simulink model "latest_coil"  (R2021b)
settings: Solver=FixedStepAuto  StartTime=-8e-3  StopTime=8e-3  FixedStep=1e-4  RelTol=1e-3
undefined symbols (not defined in the file or in its folder): X, Y, Z
libraries: sm_lib x15, nesl_utility x1
(part 1 of 2)
settings Model: Creator=teja  LastModifiedBy=teja

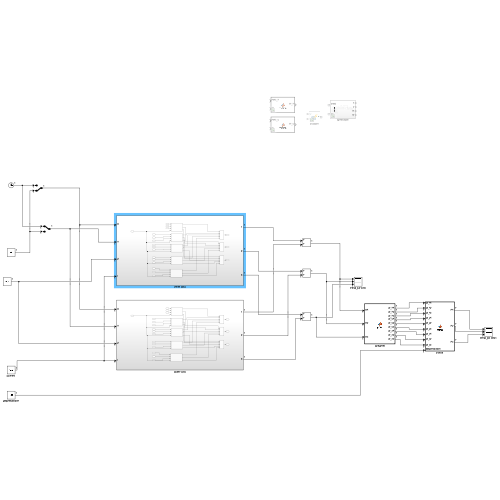
[thumbnail: Simulink's stored preview of the top-level diagram]
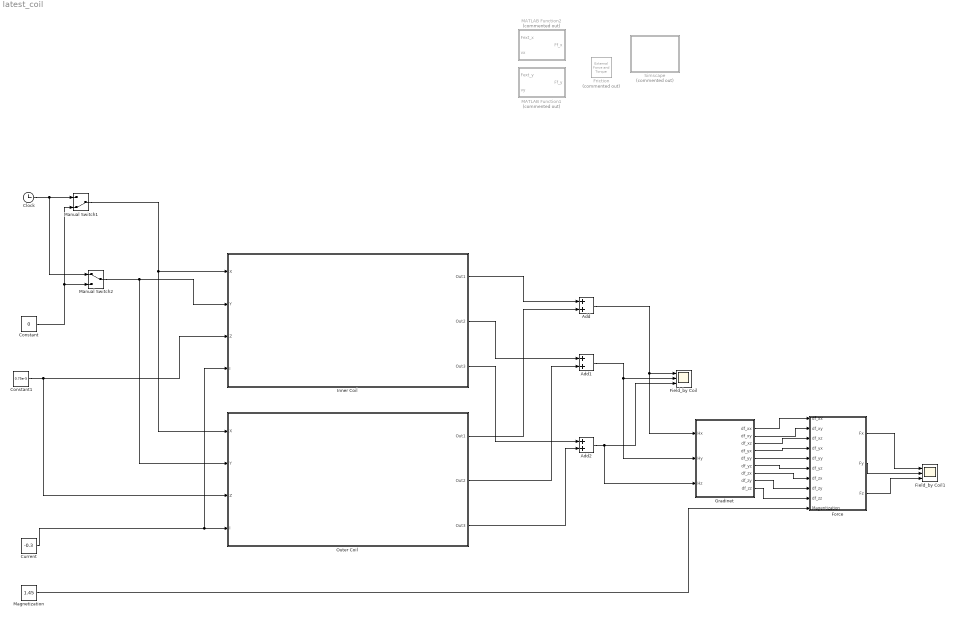
== system latest_coil ==
  Add : Sum
  Add1 : Sum
  Add2 : Sum
  Clock : Clock
  Constant : Constant  Value=0
  Constant1 : Constant  Value=0.75e-5
  Current : Constant  Value=-0.3
  Field_by Coil : Scope  NumInputPorts=3
  Field_by Coil1 : Scope  NumInputPorts=3
  Force : MATLAB Function  TreatAsAtomicUnit=on
  Friction : sm_lib/Forces and Torques/External Force and Torque  Commented=on  ForceResolutionFrame=World  EnableForceX=on  EnableForceY=on  EnableForceZ=off  EnableForce=off  TorqueResolutionFrame=AttachedFrame  EnableTorqueX=off  EnableTorqueY=off  EnableTorqueZ=off  EnableTorque=off
  Gradinet : MATLAB Function  TreatAsAtomicUnit=on
  Inner Coil : Subsystem
  MATLAB Function1 : MATLAB Function  Commented=on  TreatAsAtomicUnit=on
  MATLAB Function2 : MATLAB Function  Commented=on  TreatAsAtomicUnit=on
  Magnetization : Constant  Value=1.45
  Manual Switch1 : ManualSwitch  CurrentSetting=0
  Manual Switch2 : ManualSwitch
  Outer Coil : Subsystem
  Simscape : Subsystem  Commented=on
  wires:
  Constant/1 -> Manual Switch2/2, Manual Switch1/2
  Constant1/1 -> Outer Coil/3(Z), Inner Coil/3(Z)
  Current/1 -> Outer Coil/4(I), Inner Coil/4(I)
  Inner Coil/1(Out1) -> Add/1
  Outer Coil/1(Out1) -> Add/2
  Inner Coil/2(Out2) -> Add1/1
  Outer Coil/2(Out2) -> Add1/2
  Inner Coil/3(Out3) -> Add2/1
  Outer Coil/3(Out3) -> Add2/2
  Add2/1 -> Gradinet/3(Hz), Field_by Coil/3
  Add1/1 -> Gradinet/2(Hy), Field_by Coil/2
  Add/1 -> Gradinet/1(Hx), Field_by Coil/1
  Manual Switch1/1 -> Outer Coil/1(X), Inner Coil/1(X)
  Clock/1 -> Manual Switch2/1, Manual Switch1/1
  Manual Switch2/1 -> Outer Coil/2(Y), Inner Coil/2(Y)
  Gradinet/1(df_xx) -> Force/1(df_xx)
  Gradinet/2(df_xy) -> Force/2(df_xy)
  Gradinet/3(df_xz) -> Force/3(df_xz)
  Gradinet/4(df_yx) -> Force/4(df_yx)
  Gradinet/5(df_yy) -> Force/5(df_yy)
  Gradinet/6(df_yz) -> Force/6(df_yz)
  Gradinet/7(df_zx) -> Force/7(df_zx)
  Gradinet/8(df_zy) -> Force/8(df_zy)
  Gradinet/9(df_zz) -> Force/9(df_zz)
  Force/1(Fx) -> Field_by Coil1/1
  Force/2(Fy) -> Field_by Coil1/2
  Force/3(Fz) -> Field_by Coil1/3
  Magnetization/1 -> Force/10(Magentization)

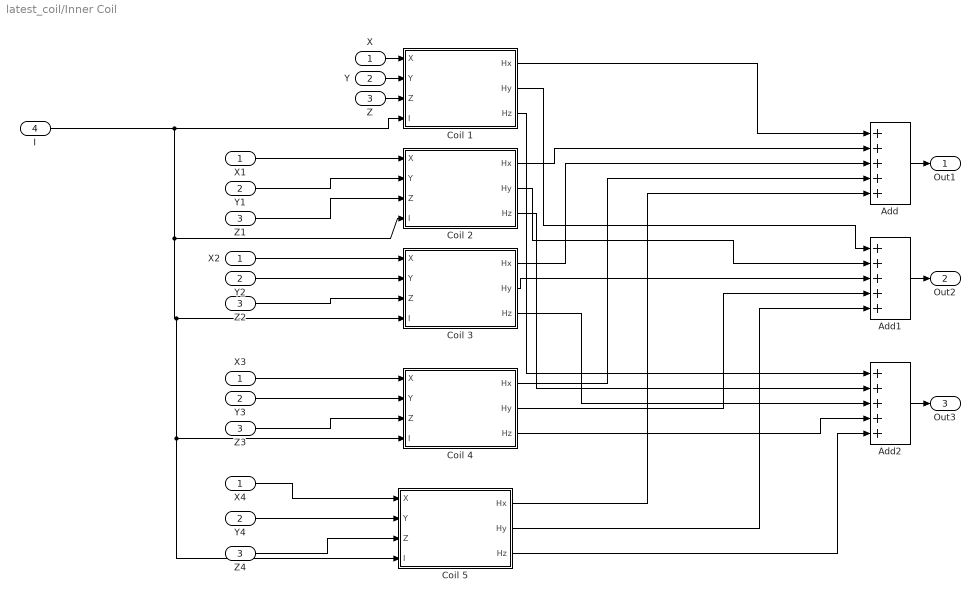
== system latest_coil/Inner Coil ==
  X : Inport
  Y : Inport  Port=2
  Z : Inport  Port=3
  I : Inport  Port=4
  Add : Sum  Inputs=+++++
  Add1 : Sum  Inputs=+++++
  Add2 : Sum  Inputs=+++++
  Coil 1 : Subsystem
  Coil 2 : Subsystem
  Coil 3 : Subsystem
  Coil 4 : Subsystem
  Coil 5 : Subsystem
  X{1..4} (4 alike) : InportShadow
  Y{1..4} (4 alike) : InportShadow  Port=2
  Z{1..4} (4 alike) : InportShadow  Port=3
  Out1 : Outport
  Out2 : Outport  Port=2
  Out3 : Outport  Port=3
  wires:
  Y/1 -> Coil 1/2(Y)
  Coil 2/2(Hy) -> Add1/2
  Add2/1 -> Out3/1
  Z/1 -> Coil 1/3(Z)
  Add1/1 -> Out2/1
  Z1/1 -> Coil 2/3(Z)
  Add/1 -> Out1/1
  Coil 4/2(Hy) -> Add1/4
  Y2/1 -> Coil 3/2(Y)
  Z2/1 -> Coil 3/3(Z)
  Coil 1/1(Hx) -> Add/1
  X4/1 -> Coil 5/1(X)
  Coil 3/2(Hy) -> Add1/3
  I/1 -> Coil 1/4(I), Coil 5/4(I), Coil 4/4(I), Coil 3/4(I), Coil 2/4(I)
  Coil 3/1(Hx) -> Add/3
  X1/1 -> Coil 2/1(X)
  Z4/1 -> Coil 5/3(Z)
  Coil 2/3(Hz) -> Add2/2
  Coil 5/2(Hy) -> Add1/5
  Coil 4/1(Hx) -> Add/4
  X3/1 -> Coil 4/1(X)
  Coil 1/2(Hy) -> Add1/1
  Coil 2/1(Hx) -> Add/2
  Z3/1 -> Coil 4/3(Z)
  Coil 5/1(Hx) -> Add/5
  Coil 3/3(Hz) -> Add2/3
  Coil 5/3(Hz) -> Add2/5
  Y4/1 -> Coil 5/2(Y)
  X/1 -> Coil 1/1(X)
  Coil 4/3(Hz) -> Add2/4
  X2/1 -> Coil 3/1(X)
  Y3/1 -> Coil 4/2(Y)
  Coil 1/3(Hz) -> Add2/1
  Y1/1 -> Coil 2/2(Y)

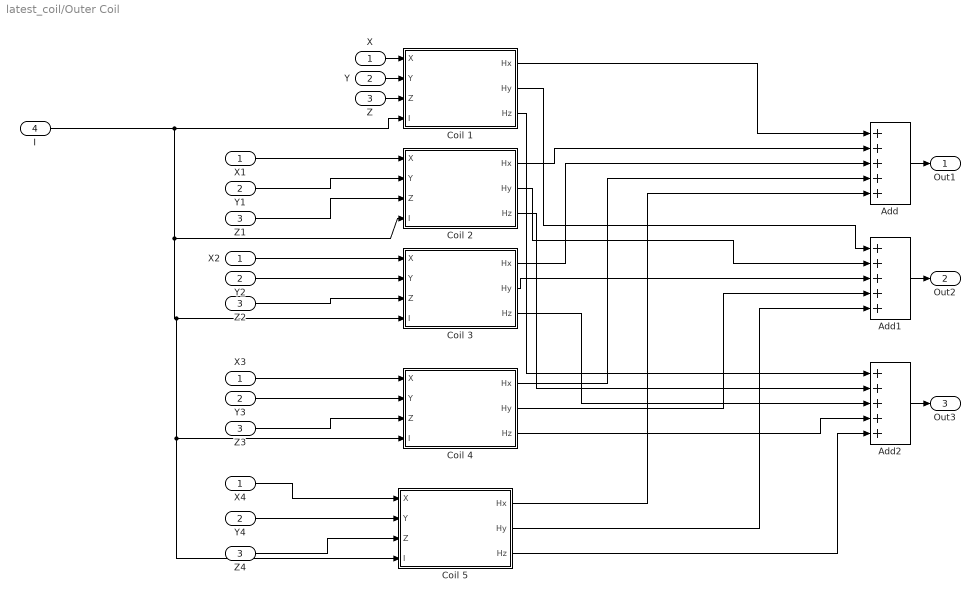
== system latest_coil/Outer Coil ==
  X : Inport
  Y : Inport  Port=2
  Z : Inport  Port=3
  I : Inport  Port=4
  Add : Sum  Inputs=+++++
  Add1 : Sum  Inputs=+++++
  Add2 : Sum  Inputs=+++++
  Coil 1 : Subsystem
  Coil 2 : Subsystem
  Coil 3 : Subsystem
  Coil 4 : Subsystem
  Coil 5 : Subsystem
  X{1..4} (4 alike) : InportShadow
  Y{1..4} (4 alike) : InportShadow  Port=2
  Z{1..4} (4 alike) : InportShadow  Port=3
  Out1 : Outport
  Out2 : Outport  Port=2
  Out3 : Outport  Port=3
  wires:
  Y1/1 -> Coil 2/2(Y)
  Coil 1/3(Hz) -> Add2/1
  Y3/1 -> Coil 4/2(Y)
  X2/1 -> Coil 3/1(X)
  Coil 4/3(Hz) -> Add2/4
  X/1 -> Coil 1/1(X)
  Y4/1 -> Coil 5/2(Y)
  Coil 5/3(Hz) -> Add2/5
  Coil 3/3(Hz) -> Add2/3
  Coil 5/1(Hx) -> Add/5
  Z3/1 -> Coil 4/3(Z)
  Coil 2/1(Hx) -> Add/2
  Coil 1/2(Hy) -> Add1/1
  X3/1 -> Coil 4/1(X)
  Coil 4/1(Hx) -> Add/4
  Coil 5/2(Hy) -> Add1/5
  Coil 2/3(Hz) -> Add2/2
  Z4/1 -> Coil 5/3(Z)
  X1/1 -> Coil 2/1(X)
  Coil 3/1(Hx) -> Add/3
  I/1 -> Coil 2/4(I), Coil 3/4(I), Coil 4/4(I), Coil 5/4(I), Coil 1/4(I)
  Coil 3/2(Hy) -> Add1/3
  X4/1 -> Coil 5/1(X)
  Coil 1/1(Hx) -> Add/1
  Z2/1 -> Coil 3/3(Z)
  Y2/1 -> Coil 3/2(Y)
  Coil 4/2(Hy) -> Add1/4
  Add/1 -> Out1/1
  Z1/1 -> Coil 2/3(Z)
  Add1/1 -> Out2/1
  Z/1 -> Coil 1/3(Z)
  Add2/1 -> Out3/1
  Coil 2/2(Hy) -> Add1/2
  Y/1 -> Coil 1/2(Y)

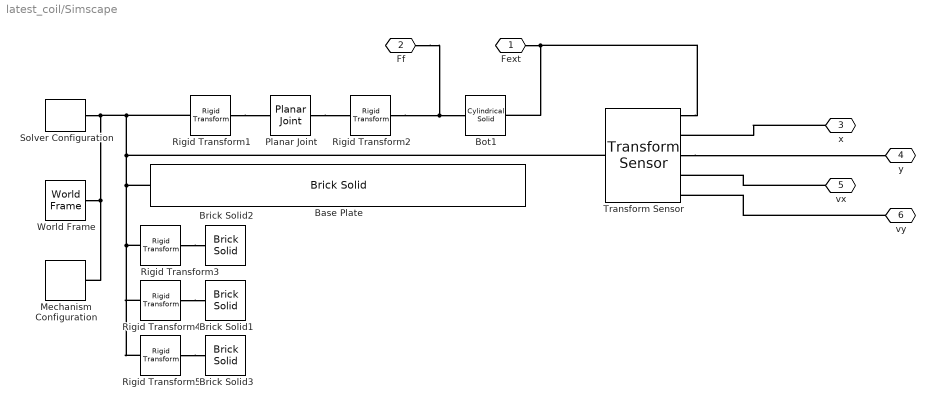
== system latest_coil/Simscape ==
  Base Plate : sm_lib/Body Elements/Brick Solid  GraphicAmbientColor=[0.15 0.15 0.15 1.0]  BasedOnType=Density  BrickDimensions=[100 100 0.15]  BrickDimensionUnits=mm  CenterOfMass=[0 0 0]  CenterOfMassUnits=m  GraphicDiffuseColor=[0.5 0.5 0.5]  Density=1000  DensityUnits=kg/m^3  DoExposeReferenceFrame=off  GraphicEmissiveColor=[0.0 0.0 0.0 1.0]  ExportEntireGeometry=off  SerializedFrames=<Frames><Frame><Id>Frame1</Id><Value><Name>Top</Name><Origin><Source>GeometricFeature</Source><FeatureName>+z surface</FeatureName></Origin><PrimaryAxis><DefinedDirection>+Z</DefinedDirection><Source>ReferenceFrame</Source><SourceDirection>+Z</SourceDirection><FeatureName></FeatureName></PrimaryAxis><SecondaryAxis><DefinedDirection>+X</DefinedDirection><Source>ReferenceFrame</Source><SourceDirection>+X</SourceDirection><FeatureName></FeatureName></SecondaryAxis></Value></Frame></Frames>  MarkerShape=Sphere  MarkerSize=10  GraphicType=FromGeometry  InertiaType=CalculateFromGeometry  Mass=1  MassUnits=kg  MomentsOfInertia=[1 1 1]  MomentsOfInertiaUnits=kg*m^2  GraphicOpacity=1.0  ProductsOfInertia=[0 0 0]  ProductsOfInertiaUnits=kg*m^2  GraphicShininess=75  GraphicSpecularColor=[0.5 0.5 0.5 1.0]  GraphicVisPropType=SimpleVisualProperties
  Bot1 : sm_lib/Body Elements/Cylindrical Solid  GraphicAmbientColor=[0.15 0.15 0.15 1.0]  BasedOnType=Density  CenterOfMass=[0 0 0]  CenterOfMassUnits=m  GraphicDiffuseColor=[0 0.5 0.5]  CylinderLength=10  CylinderLengthUnits=mm  CylinderRadius=20  CylinderRadiusUnits=mm  Density=7300  DensityUnits=kg/m^3  DoExposeReferenceFrame=on  GraphicEmissiveColor=[0.0 0.0 0.0 1.0]  ExportEntireGeometry=off  SerializedFrames=<Frames><Frame><Id>Frame1</Id><Value><Name>Bottom</Name><Origin><Source>GeometricFeature</Source><FeatureName>bottom surface</FeatureName></Origin><PrimaryAxis><DefinedDirection>+Z</DefinedDirection><Source>ReferenceFrame</Source><SourceDirection>+Z</SourceDirection><FeatureName></FeatureName></PrimaryAxis><SecondaryAxis><DefinedDirection>+X</DefinedDirection><Source>ReferenceFrame</Source><SourceDirection>+X</SourceDirection><FeatureName></FeatureName></SecondaryAxis></Value></Frame></Frames>  MarkerShape=Sphere  MarkerSize=10  GraphicType=FromGeometry  InertiaType=CalculateFromGeometry  Mass=1  MassUnits=kg  MomentsOfInertia=[1 1 1]  MomentsOfInertiaUnits=kg*m^2  GraphicOpacity=1.0  ProductsOfInertia=[0 0 0]  ProductsOfInertiaUnits=kg*m^2  GraphicShininess=75  GraphicSpecularColor=[0.5 0.5 0.5 1.0]  GraphicVisPropType=SimpleVisualProperties
  Brick Solid1 : sm_lib/Body Elements/Brick Solid  GraphicAmbientColor=[0.15 0.15 0.15 1.0]  BasedOnType=Density  BrickDimensions=[8 8 0.5]  BrickDimensionUnits=mm  CenterOfMass=[0 0 0]  CenterOfMassUnits=m  GraphicDiffuseColor=[0.5 0.5 0]  Density=1000  DensityUnits=kg/m^3  DoExposeReferenceFrame=off  GraphicEmissiveColor=[0.0 0.0 0.0 1.0]  ExportEntireGeometry=off  SerializedFrames=<Frames><Frame><Id>Frame1</Id><Value><Name>base</Name><Origin><Source>GeometricFeature</Source><FeatureName>-z surface</FeatureName></Origin><PrimaryAxis><DefinedDirection>+Z</DefinedDirection><Source>ReferenceFrame</Source><SourceDirection>+Z</SourceDirection><FeatureName></FeatureName></PrimaryAxis><SecondaryAxis><DefinedDirection>+X</DefinedDirection><Source>ReferenceFrame</Source><SourceDirection>+X</SourceDirection><FeatureName></FeatureName></SecondaryAxis></Value></Frame></Frames>  MarkerShape=Sphere  MarkerSize=10  GraphicType=FromGeometry  InertiaType=CalculateFromGeometry  Mass=1  MassUnits=kg  MomentsOfInertia=[1 1 1]  MomentsOfInertiaUnits=kg*m^2  GraphicOpacity=1.0  ProductsOfInertia=[0 0 0]  ProductsOfInertiaUnits=kg*m^2  GraphicShininess=75  GraphicSpecularColor=[0.5 0.5 0.5 1.0]  GraphicVisPropType=SimpleVisualProperties
  Brick Solid2 : sm_lib/Body Elements/Brick Solid  GraphicAmbientColor=[0.15 0.15 0.15 1.0]  BasedOnType=Density  BrickDimensions=[8 8 0.5]  BrickDimensionUnits=mm  CenterOfMass=[0 0 0]  CenterOfMassUnits=m  GraphicDiffuseColor=[0.5 0.5 0]  Density=1000  DensityUnits=kg/m^3  DoExposeReferenceFrame=off  GraphicEmissiveColor=[0.0 0.0 0.0 1.0]  ExportEntireGeometry=off  SerializedFrames=<Frames><Frame><Id>Frame1</Id><Value><Name>base</Name><Origin><Source>GeometricFeature</Source><FeatureName>-z surface</FeatureName></Origin><PrimaryAxis><DefinedDirection>+Z</DefinedDirection><Source>ReferenceFrame</Source><SourceDirection>+Z</SourceDirection><FeatureName></FeatureName></PrimaryAxis><SecondaryAxis><DefinedDirection>+X</DefinedDirection><Source>ReferenceFrame</Source><SourceDirection>+X</SourceDirection><FeatureName></FeatureName></SecondaryAxis></Value></Frame></Frames>  MarkerShape=Sphere  MarkerSize=10  GraphicType=FromGeometry  InertiaType=CalculateFromGeometry  Mass=1  MassUnits=kg  MomentsOfInertia=[1 1 1]  MomentsOfInertiaUnits=kg*m^2  GraphicOpacity=1.0  ProductsOfInertia=[0 0 0]  ProductsOfInertiaUnits=kg*m^2  GraphicShininess=75  GraphicSpecularColor=[0.5 0.5 0.5 1.0]  GraphicVisPropType=SimpleVisualProperties
  Brick Solid3 : sm_lib/Body Elements/Brick Solid  GraphicAmbientColor=[0.15 0.15 0.15 1.0]  BasedOnType=Density  BrickDimensions=[8 8 0.5]  BrickDimensionUnits=mm  CenterOfMass=[0 0 0]  CenterOfMassUnits=m  GraphicDiffuseColor=[0.5 0.5 0]  Density=1000  DensityUnits=kg/m^3  DoExposeReferenceFrame=off  GraphicEmissiveColor=[0.0 0.0 0.0 1.0]  ExportEntireGeometry=off  SerializedFrames=<Frames><Frame><Id>Frame1</Id><Value><Name>base</Name><Origin><Source>GeometricFeature</Source><FeatureName>-z surface</FeatureName></Origin><PrimaryAxis><DefinedDirection>+Z</DefinedDirection><Source>ReferenceFrame</Source><SourceDirection>+Z</SourceDirection><FeatureName></FeatureName></PrimaryAxis><SecondaryAxis><DefinedDirection>+X</DefinedDirection><Source>ReferenceFrame</Source><SourceDirection>+X</SourceDirection><FeatureName></FeatureName></SecondaryAxis></Value></Frame></Frames>  MarkerShape=Sphere  MarkerSize=10  GraphicType=FromGeometry  InertiaType=CalculateFromGeometry  Mass=1  MassUnits=kg  MomentsOfInertia=[1 1 1]  MomentsOfInertiaUnits=kg*m^2  GraphicOpacity=1.0  ProductsOfInertia=[0 0 0]  ProductsOfInertiaUnits=kg*m^2  GraphicShininess=75  GraphicSpecularColor=[0.5 0.5 0.5 1.0]  GraphicVisPropType=SimpleVisualProperties
  Mechanism Configuration : sm_lib/Utilities/Mechanism Configuration  UniformGravity=Constant  GravityVector=[0 0 -9.80665]  GravityUnits=m/s^2  LinearizationDelta=0.001  JointModeTransitionNonlinearIterations=2
  Planar Joint : sm_lib/Joints/Planar Joint  JointMode=Normal  SenseConstraintForce=off  SenseConstraintForceX=off  SenseConstraintForceY=off  SenseConstraintForceZ=off  SenseConstraintTorque=off  SenseConstraintTorqueX=off  SenseConstraintTorqueY=off  SenseConstraintTorqueZ=off  SenseTotalForce=off  SenseTotalForceX=off  SenseTotalForceY=off  SenseTotalForceZ=off  SenseTotalTorque=off  SenseTotalTorqueX=off  SenseTotalTorqueY=off  SenseTotalTorqueZ=off  CompositeWrenchDir=FollowerOnBase  CompositeWrenchFrame=BaseFrame  PxEquilibriumPosition=0  PxEquilibriumPositionUnits=m  PxSpringStiffness=0  PxSpringStiffnessUnits=N/m  PxDampingCoefficient=0  PxDampingCoefficientUnits=N/(m/s)  PxTorqueActuationMode=NoTorque  PxMotionActuationMode=ComputedMotion  PxSensePosition=off  PxSenseVelocity=off  PxSenseAcceleration=off  PxSenseTorqueForce=off  PxSenseLowerLimitTorqueForce=off  PxSenseUpperLimitTorqueForce=off  PxLowerLimitSpecify=off  PxLowerLimitBound=-1  PxLowerLimitBoundUnits=m  PxLowerLimitStiffness=1e6  PxLowerLimitStiffnessUnits=N/m  PxLowerLimitDamping=1e3  PxLowerLimitDampingUnits=N/(m/s)  PxLowerLimitTransitionRegionWidth=1e-4  PxLowerLimitTransitionRegionWidthUnits=m  PxUpperLimitSpecify=off  PxUpperLimitBound=1  PxUpperLimitBoundUnits=m  PxUpperLimitStiffness=1e6  PxUpperLimitStiffnessUnits=N/m  PxUpperLimitDamping=1e3  PxUpperLimitDampingUnits=N/(m/s)  PxUpperLimitTransitionRegionWidth=1e-4  PxUpperLimitTransitionRegionWidthUnits=m  PxPositionTargetSpecify=off  PxPositionTargetPriority=High  PxPositionTargetValue=0  PxPositionTargetValueUnits=m  PxVelocityTargetSpecify=off  PxVelocityTargetPriority=High  PxVelocityTargetValue=0  PxVelocityTargetValueUnits=m/s  PyEquilibriumPosition=0  PyEquilibriumPositionUnits=m  PySpringStiffness=0  PySpringStiffnessUnits=N/m  PyDampingCoefficient=0  PyDampingCoefficientUnits=N/(m/s)  PyTorqueActuationMode=NoTorque  PyMotionActuationMode=ComputedMotion  PySensePosition=off  PySenseVelocity=off  PySenseAcceleration=off  PySenseTorqueForce=off  PySenseLowerLimitTorqueForce=off  PySenseUpperLimitTorqueForce=off  PyLowerLimitSpecify=off  PyLowerLimitBound=-1  PyLowerLimitBoundUnits=m  PyLowerLimitStiffness=1e6  PyLowerLimitStiffnessUnits=N/m  PyLowerLimitDamping=1e3  PyLowerLimitDampingUnits=N/(m/s)  PyLowerLimitTransitionRegionWidth=1e-4  PyLowerLimitTransitionRegionWidthUnits=m  PyUpperLimitSpecify=off  PyUpperLimitBound=1  PyUpperLimitBoundUnits=m  PyUpperLimitStiffness=1e6  PyUpperLimitStiffnessUnits=N/m  PyUpperLimitDamping=1e3  PyUpperLimitDampingUnits=N/(m/s)  PyUpperLimitTransitionRegionWidth=1e-4  PyUpperLimitTransitionRegionWidthUnits=m  PyPositionTargetSpecify=off  PyPositionTargetPriority=High  PyPositionTargetValue=0  PyPositionTargetValueUnits=m  PyVelocityTargetSpecify=off  PyVelocityTargetPriority=High  PyVelocityTargetValue=0  PyVelocityTargetValueUnits=m/s  RzEquilibriumPosition=0  RzEquilibriumPositionUnits=deg  RzSpringStiffness=0  RzSpringStiffnessUnits=N*m/deg  RzDampingCoefficient=0  RzDampingCoefficientUnits=N*m/(deg/s)  RzTorqueActuationMode=NoTorque  RzMotionActuationMode=ComputedMotion  RzSensePosition=off  RzSenseVelocity=off  RzSenseAcceleration=off  RzSenseTorqueForce=off  RzSenseLowerLimitTorqueForce=off  RzSenseUpperLimitTorqueForce=off  RzLowerLimitSpecify=off  RzLowerLimitBound=-90  RzLowerLimitBoundUnits=deg  RzLowerLimitStiffness=1e4  RzLowerLimitStiffnessUnits=N*m/deg  RzLowerLimitDamping=10  RzLowerLimitDampingUnits=N*m/(deg/s)  RzLowerLimitTransitionRegionWidth=0.1  RzLowerLimitTransitionRegionWidthUnits=deg  RzUpperLimitSpecify=off  RzUpperLimitBound=90  RzUpperLimitBoundUnits=deg  RzUpperLimitStiffness=1e4  RzUpperLimitStiffnessUnits=N*m/deg  RzUpperLimitDamping=10  RzUpperLimitDampingUnits=N*m/(deg/s)  RzUpperLimitTransitionRegionWidth=0.1  RzUpperLimitTransitionRegionWidthUnits=deg  RzPositionTargetSpecify=off  RzPositionTargetPriority=High  RzPositionTargetValue=0  RzPositionTargetValueUnits=deg  RzVelocityTargetSpecify=off  RzVelocityTargetPriority=High  RzVelocityTargetValue=0  RzVelocityTargetValueUnits=deg/s
  Rigid Transform1 : sm_lib/Frames and Transforms/Rigid Transform  TranslationMethod=Cartesian  TranslationStandardOffset=0  TranslationLengthUnit=mm  TranslationStandardAxis=+Z  TranslationCartesianOffset=[0 0 0]  TranslationROffset=0  TranslationROffsetUnits=m  TranslationZOffset=0  TranslationZOffsetUnits=m  TranslationThetaOffset=0  TranslationThetaOffsetUnits=deg  RotationMethod=AlignedAxes  RotationAngleUnits=deg  RotationStandardAxis=+Z  RotationAngle=0.0  RotationArbitraryAxis=[0 0 1]  FollAlignAxisA=+Y  BaseAlignAxisA=+X  FollAlignAxisB=+Z  BaseAlignAxisB=+Z  RotationSequenceAxes=FollowerAxes  RotationSequence=XYX  RotationSequenceAngles=[0 0 0]  RotationSequenceAnglesUnits=deg  RotationMatrix=[1 0 0; 0 1 0; 0 0 1]
  Rigid Transform2 : sm_lib/Frames and Transforms/Rigid Transform  TranslationMethod=None  TranslationStandardOffset=0  TranslationLengthUnit=mm  TranslationStandardAxis=+Z  TranslationCartesianOffset=[-15 0 0.15]  TranslationROffset=0  TranslationROffsetUnits=m  TranslationZOffset=0  TranslationZOffsetUnits=m  TranslationThetaOffset=0  TranslationThetaOffsetUnits=deg  RotationMethod=AlignedAxes  RotationAngleUnits=deg  RotationStandardAxis=+Z  RotationAngle=0.0  RotationArbitraryAxis=[0 0 1]  FollAlignAxisA=+Y  BaseAlignAxisA=+X  FollAlignAxisB=+Z  BaseAlignAxisB=+Z  RotationSequenceAxes=FollowerAxes  RotationSequence=XYX  RotationSequenceAngles=[0 0 0]  RotationSequenceAnglesUnits=deg  RotationMatrix=[1 0 0; 0 1 0; 0 0 1]
  Rigid Transform3 : sm_lib/Frames and Transforms/Rigid Transform  TranslationMethod=Cartesian  TranslationStandardOffset=0  TranslationLengthUnit=mm  TranslationStandardAxis=+Z  TranslationCartesianOffset=[9 0 2]  TranslationROffset=0  TranslationROffsetUnits=m  TranslationZOffset=0  TranslationZOffsetUnits=m  TranslationThetaOffset=0  TranslationThetaOffsetUnits=deg  RotationMethod=None  RotationAngleUnits=deg  RotationStandardAxis=+Z  RotationAngle=0.0  RotationArbitraryAxis=[0 0 1]  FollAlignAxisA=+Y  BaseAlignAxisA=+X  FollAlignAxisB=+Z  BaseAlignAxisB=+Z  RotationSequenceAxes=FollowerAxes  RotationSequence=XYX  RotationSequenceAngles=[0 0 0]  RotationSequenceAnglesUnits=deg  RotationMatrix=[1 0 0; 0 1 0; 0 0 1]
  Rigid Transform4 : sm_lib/Frames and Transforms/Rigid Transform  TranslationMethod=Cartesian  TranslationStandardOffset=0  TranslationLengthUnit=mm  TranslationStandardAxis=+Z  TranslationCartesianOffset=[0 0 2]  TranslationROffset=0  TranslationROffsetUnits=m  TranslationZOffset=0  TranslationZOffsetUnits=m  TranslationThetaOffset=0  TranslationThetaOffsetUnits=deg  RotationMethod=None  RotationAngleUnits=deg  RotationStandardAxis=+Z  RotationAngle=0.0  RotationArbitraryAxis=[0 0 1]  FollAlignAxisA=+Y  BaseAlignAxisA=+X  FollAlignAxisB=+Z  BaseAlignAxisB=+Z  RotationSequenceAxes=FollowerAxes  RotationSequence=XYX  RotationSequenceAngles=[0 0 0]  RotationSequenceAnglesUnits=deg  RotationMatrix=[1 0 0; 0 1 0; 0 0 1]
  Rigid Transform5 : sm_lib/Frames and Transforms/Rigid Transform  TranslationMethod=Cartesian  TranslationStandardOffset=0  TranslationLengthUnit=mm  TranslationStandardAxis=+Z  TranslationCartesianOffset=[-9 0 2]  TranslationROffset=0  TranslationROffsetUnits=m  TranslationZOffset=0  TranslationZOffsetUnits=m  TranslationThetaOffset=0  TranslationThetaOffsetUnits=deg  RotationMethod=None  RotationAngleUnits=deg  RotationStandardAxis=+Z  RotationAngle=0.0  RotationArbitraryAxis=[0 0 1]  FollAlignAxisA=+Y  BaseAlignAxisA=+X  FollAlignAxisB=+Z  BaseAlignAxisB=+Z  RotationSequenceAxes=FollowerAxes  RotationSequence=XYX  RotationSequenceAngles=[0 0 0]  RotationSequenceAnglesUnits=deg  RotationMatrix=[1 0 0; 0 1 0; 0 0 1]
  Solver Configuration : nesl_utility/Solver Configuration  PhysicalDomain=network_engine_domain  SubClassName=solver  LeftPortType=input  RightPortType=generic  Tones=[]  Harmonics=[]  SimulateNoise=off  Profile=off  UseLocalSampling=off  EnableSwitchedLinearOptims=on  FrequencyDomain=off  UseCCode=off  RelTol=0.001  AbsTol=1e-06  MinStep=1e-09  ToWorkspace=off  RevertToSquareIcSolve=off  NumHomotopyIterations=100  PhasorMode=off  PhasorModeNumHarmonics=1  DoDC=off  ResidualTolerance=1e-09  UseLocalSolver=off  LocalSolverChoice=NE_BACKWARD_EULER_ADVANCER  LocalSolverSampleTime=0.001  DoFixedCost=off  MaxNonlinIter=3  MaxModeIter=2  ComputeImpulses=off  ImpulseIterations=2  LinearAlgebra=Sparse  EquationFormulation=NE_TIME_EF  DelaysMemoryBudget=1024  AutomaticFiltering=on  FilteringTimeConstant=0.001  PartitionStorageMethod=AS_NEEDED  PartitionMemoryBudget=1024  PartitionMethod=FAST
      settings: SourceProductBaseCode=PW,SS
  Transform Sensor : sm_lib/Frames and Transforms/Transform Sensor  MeasurementFrame=World  SenseAngle=off  SenseAxis=off  SenseAngle1=off  SenseAngle2=off  SenseAngle3=off  SenseQ=off  SenseR=off  SenseOmegaX=off  SenseOmegaY=off  SenseOmegaZ=off  SenseOmega1=off  SenseOmega2=off  SenseOmega3=off  SenseQDot=off  SenseRDot=off  SenseAlphaX=off  SenseAlphaY=off  SenseAlphaZ=off  SenseAlpha1=off  SenseAlpha2=off  SenseAlpha3=off  SenseQDDot=off  SenseRDDot=off  SenseX=on  SenseY=on  SenseZ=off  SenseRad=off  SenseAzim=off  SenseDist=off  SenseInc=off  SenseXDot=on  SenseYDot=on  SenseZDot=off  SenseRadDot=off  SenseAzimDot=off  SenseDistDot=off  SenseIncDot=off  SenseXDDot=off  SenseYDDot=off  SenseZDDot=off  SenseRadDDot=off  SenseAzimDDot=off  SenseDistDDot=off  SenseIncDDot=off
  World Frame : sm_lib/Frames and Transforms/World Frame
  Fext : PMIOPort  Side=Left
  Ff : PMIOPort  Port=2  Side=Left
  x : PMIOPort  Port=3  Side=Right
  y : PMIOPort  Port=4  Side=Right
  vx : PMIOPort  Port=5  Side=Right
  vy : PMIOPort  Port=6  Side=Right
  connections:
  Rigid Transform1/RConn1 -- Planar Joint/LConn1
  Rigid Transform4/RConn1 -- Brick Solid1/LConn1
  Planar Joint/RConn1 -- Rigid Transform2/LConn1
  Rigid Transform2/RConn1 -- Ff/RConn1 -- Bot1/LConn1
  x/RConn1 -- Transform Sensor/RConn2
  Transform Sensor/RConn3 -- y/RConn1
  vy/RConn1 -- Transform Sensor/RConn5
  vx/RConn1 -- Transform Sensor/RConn4
  Solver Configuration/RConn1 -- Mechanism Configuration/RConn1 -- World Frame/RConn1 -- Transform Sensor/LConn1 -- Rigid Transform5/LConn1 -- Rigid Transform4/LConn1 -- Rigid Transform3/LConn1 -- Base Plate/LConn1 -- Rigid Transform1/LConn1
  Transform Sensor/RConn1 -- Fext/RConn1 -- Bot1/RConn1
  Rigid Transform3/RConn1 -- Brick Solid2/LConn1
  Rigid Transform5/RConn1 -- Brick Solid3/LConn1

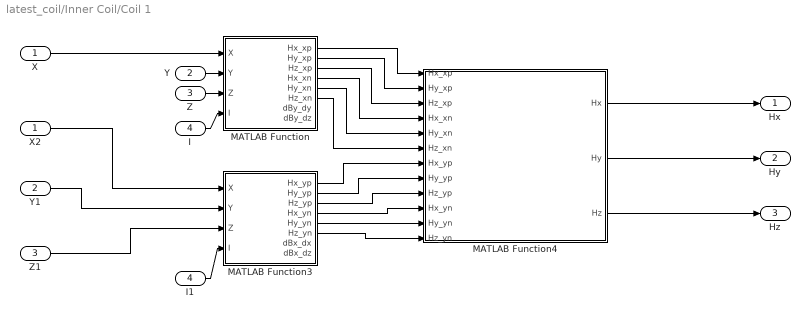
== system latest_coil/Inner Coil/Coil 1 ==
  X : Inport
  Y : Inport  Port=2
  Z : Inport  Port=3
  I : Inport  Port=4
  I1 : InportShadow  Port=4
  MATLAB Function : MATLAB Function  TreatAsAtomicUnit=on
  MATLAB Function3 : MATLAB Function  TreatAsAtomicUnit=on
  MATLAB Function4 : MATLAB Function  TreatAsAtomicUnit=on
  X2 : InportShadow
  Y1 : InportShadow  Port=2
  Z1 : InportShadow  Port=3
  Hx : Outport
  Hy : Outport  Port=2
  Hz : Outport  Port=3
  wires:
  MATLAB Function4/3(Hz) -> Hz/1
  X/1 -> MATLAB Function/1(X)
  MATLAB Function4/1(Hx) -> Hx/1
  I1/1 -> MATLAB Function3/4(I)
  MATLAB Function/6(Hz_xn) -> MATLAB Function4/6(Hz_xn)
  Z/1 -> MATLAB Function/3(Z)
  MATLAB Function/3(Hz_xp) -> MATLAB Function4/3(Hz_xp)
  MATLAB Function4/2(Hy) -> Hy/1
  MATLAB Function3/1(Hx_yp) -> MATLAB Function4/7(Hx_yp)
  MATLAB Function3/4(Hx_yn) -> MATLAB Function4/10(Hx_yn)
  MATLAB Function3/3(Hz_yp) -> MATLAB Function4/9(Hz_yp)
  MATLAB Function/4(Hx_xn) -> MATLAB Function4/4(Hx_xn)
  MATLAB Function/1(Hx_xp) -> MATLAB Function4/1(Hx_xp)
  MATLAB Function3/2(Hy_yp) -> MATLAB Function4/8(Hy_yp)
  Y/1 -> MATLAB Function/2(Y)
  MATLAB Function/5(Hy_xn) -> MATLAB Function4/5(Hy_xn)
  MATLAB Function3/5(Hy_yn) -> MATLAB Function4/11(Hy_yn)
  MATLAB Function3/6(Hz_yn) -> MATLAB Function4/12(Hz_yn)
  MATLAB Function/2(Hy_xp) -> MATLAB Function4/2(Hy_xp)
  I/1 -> MATLAB Function/4(I)
  X2/1 -> MATLAB Function3/1(X)
  Y1/1 -> MATLAB Function3/2(Y)
  Z1/1 -> MATLAB Function3/3(Z)

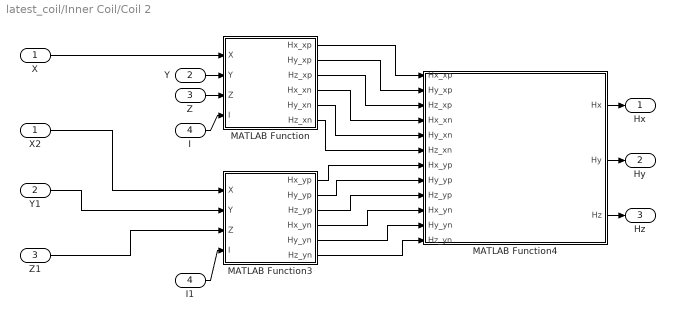
== system latest_coil/Inner Coil/Coil 2 ==
  X : Inport
  Y : Inport  Port=2
  Z : Inport  Port=3
  I : Inport  Port=4
  I1 : InportShadow  Port=4
  MATLAB Function : MATLAB Function  TreatAsAtomicUnit=on
  MATLAB Function3 : MATLAB Function  TreatAsAtomicUnit=on
  MATLAB Function4 : MATLAB Function  TreatAsAtomicUnit=on
  X2 : InportShadow
  Y1 : InportShadow  Port=2
  Z1 : InportShadow  Port=3
  Hx : Outport
  Hy : Outport  Port=2
  Hz : Outport  Port=3
  wires:
  Z1/1 -> MATLAB Function3/3(Z)
  Y1/1 -> MATLAB Function3/2(Y)
  X2/1 -> MATLAB Function3/1(X)
  I/1 -> MATLAB Function/4(I)
  MATLAB Function/2(Hy_xp) -> MATLAB Function4/2(Hy_xp)
  MATLAB Function3/6(Hz_yn) -> MATLAB Function4/12(Hz_yn)
  MATLAB Function3/5(Hy_yn) -> MATLAB Function4/11(Hy_yn)
  MATLAB Function/5(Hy_xn) -> MATLAB Function4/5(Hy_xn)
  Y/1 -> MATLAB Function/2(Y)
  MATLAB Function3/2(Hy_yp) -> MATLAB Function4/8(Hy_yp)
  MATLAB Function/1(Hx_xp) -> MATLAB Function4/1(Hx_xp)
  MATLAB Function/4(Hx_xn) -> MATLAB Function4/4(Hx_xn)
  MATLAB Function3/3(Hz_yp) -> MATLAB Function4/9(Hz_yp)
  MATLAB Function3/4(Hx_yn) -> MATLAB Function4/10(Hx_yn)
  MATLAB Function3/1(Hx_yp) -> MATLAB Function4/7(Hx_yp)
  MATLAB Function4/2(Hy) -> Hy/1
  MATLAB Function/3(Hz_xp) -> MATLAB Function4/3(Hz_xp)
  Z/1 -> MATLAB Function/3(Z)
  MATLAB Function/6(Hz_xn) -> MATLAB Function4/6(Hz_xn)
  I1/1 -> MATLAB Function3/4(I)
  MATLAB Function4/1(Hx) -> Hx/1
  X/1 -> MATLAB Function/1(X)
  MATLAB Function4/3(Hz) -> Hz/1

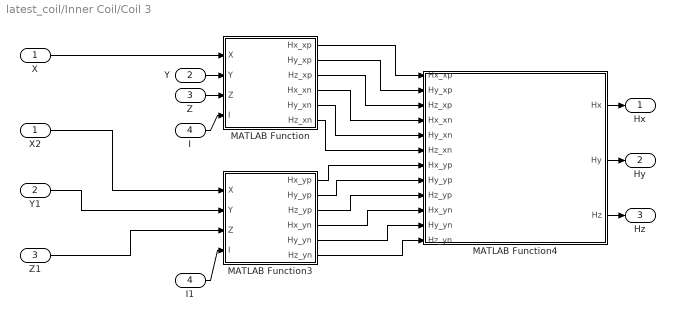
== system latest_coil/Inner Coil/Coil 3 ==
  X : Inport
  Y : Inport  Port=2
  Z : Inport  Port=3
  I : Inport  Port=4
  I1 : InportShadow  Port=4
  MATLAB Function : MATLAB Function  TreatAsAtomicUnit=on
  MATLAB Function3 : MATLAB Function  TreatAsAtomicUnit=on
  MATLAB Function4 : MATLAB Function  TreatAsAtomicUnit=on
  X2 : InportShadow
  Y1 : InportShadow  Port=2
  Z1 : InportShadow  Port=3
  Hx : Outport
  Hy : Outport  Port=2
  Hz : Outport  Port=3
  wires:
  Z1/1 -> MATLAB Function3/3(Z)
  Y1/1 -> MATLAB Function3/2(Y)
  X2/1 -> MATLAB Function3/1(X)
  I/1 -> MATLAB Function/4(I)
  MATLAB Function/2(Hy_xp) -> MATLAB Function4/2(Hy_xp)
  MATLAB Function3/6(Hz_yn) -> MATLAB Function4/12(Hz_yn)
  MATLAB Function3/5(Hy_yn) -> MATLAB Function4/11(Hy_yn)
  MATLAB Function/5(Hy_xn) -> MATLAB Function4/5(Hy_xn)
  Y/1 -> MATLAB Function/2(Y)
  MATLAB Function3/2(Hy_yp) -> MATLAB Function4/8(Hy_yp)
  MATLAB Function/1(Hx_xp) -> MATLAB Function4/1(Hx_xp)
  MATLAB Function/4(Hx_xn) -> MATLAB Function4/4(Hx_xn)
  MATLAB Function3/3(Hz_yp) -> MATLAB Function4/9(Hz_yp)
  MATLAB Function3/4(Hx_yn) -> MATLAB Function4/10(Hx_yn)
  MATLAB Function3/1(Hx_yp) -> MATLAB Function4/7(Hx_yp)
  MATLAB Function4/2(Hy) -> Hy/1
  MATLAB Function/3(Hz_xp) -> MATLAB Function4/3(Hz_xp)
  Z/1 -> MATLAB Function/3(Z)
  MATLAB Function/6(Hz_xn) -> MATLAB Function4/6(Hz_xn)
  I1/1 -> MATLAB Function3/4(I)
  MATLAB Function4/1(Hx) -> Hx/1
  X/1 -> MATLAB Function/1(X)
  MATLAB Function4/3(Hz) -> Hz/1

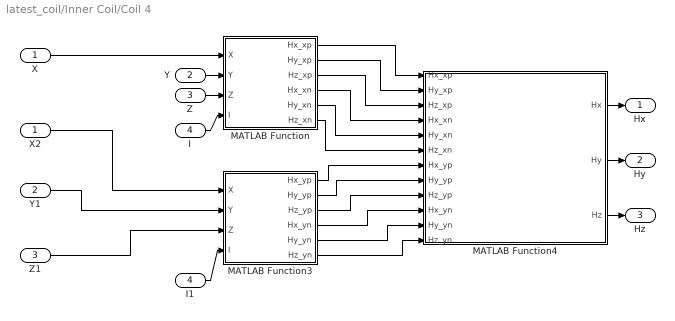
== system latest_coil/Inner Coil/Coil 4 ==
  X : Inport
  Y : Inport  Port=2
  Z : Inport  Port=3
  I : Inport  Port=4
  I1 : InportShadow  Port=4
  MATLAB Function : MATLAB Function  TreatAsAtomicUnit=on
  MATLAB Function3 : MATLAB Function  TreatAsAtomicUnit=on
  MATLAB Function4 : MATLAB Function  TreatAsAtomicUnit=on
  X2 : InportShadow
  Y1 : InportShadow  Port=2
  Z1 : InportShadow  Port=3
  Hx : Outport
  Hy : Outport  Port=2
  Hz : Outport  Port=3
  wires:
  MATLAB Function4/3(Hz) -> Hz/1
  X/1 -> MATLAB Function/1(X)
  MATLAB Function4/1(Hx) -> Hx/1
  I1/1 -> MATLAB Function3/4(I)
  MATLAB Function/6(Hz_xn) -> MATLAB Function4/6(Hz_xn)
  Z/1 -> MATLAB Function/3(Z)
  MATLAB Function/3(Hz_xp) -> MATLAB Function4/3(Hz_xp)
  MATLAB Function4/2(Hy) -> Hy/1
  MATLAB Function3/1(Hx_yp) -> MATLAB Function4/7(Hx_yp)
  MATLAB Function3/4(Hx_yn) -> MATLAB Function4/10(Hx_yn)
  MATLAB Function3/3(Hz_yp) -> MATLAB Function4/9(Hz_yp)
  MATLAB Function/4(Hx_xn) -> MATLAB Function4/4(Hx_xn)
  MATLAB Function/1(Hx_xp) -> MATLAB Function4/1(Hx_xp)
  MATLAB Function3/2(Hy_yp) -> MATLAB Function4/8(Hy_yp)
  Y/1 -> MATLAB Function/2(Y)
  MATLAB Function/5(Hy_xn) -> MATLAB Function4/5(Hy_xn)
  MATLAB Function3/5(Hy_yn) -> MATLAB Function4/11(Hy_yn)
  MATLAB Function3/6(Hz_yn) -> MATLAB Function4/12(Hz_yn)
  MATLAB Function/2(Hy_xp) -> MATLAB Function4/2(Hy_xp)
  I/1 -> MATLAB Function/4(I)
  X2/1 -> MATLAB Function3/1(X)
  Y1/1 -> MATLAB Function3/2(Y)
  Z1/1 -> MATLAB Function3/3(Z)

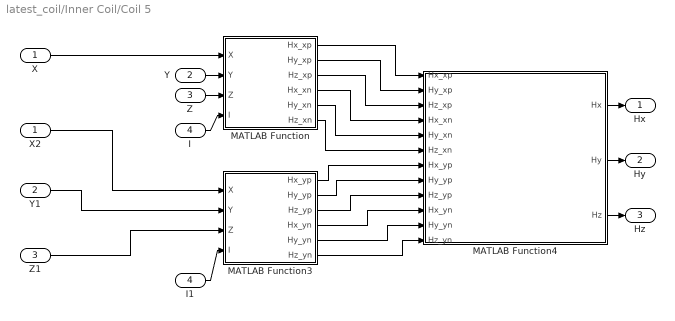
== system latest_coil/Inner Coil/Coil 5 ==
  X : Inport
  Y : Inport  Port=2
  Z : Inport  Port=3
  I : Inport  Port=4
  I1 : InportShadow  Port=4
  MATLAB Function : MATLAB Function  TreatAsAtomicUnit=on
  MATLAB Function3 : MATLAB Function  TreatAsAtomicUnit=on
  MATLAB Function4 : MATLAB Function  TreatAsAtomicUnit=on
  X2 : InportShadow
  Y1 : InportShadow  Port=2
  Z1 : InportShadow  Port=3
  Hx : Outport
  Hy : Outport  Port=2
  Hz : Outport  Port=3
  wires:
  Z1/1 -> MATLAB Function3/3(Z)
  Y1/1 -> MATLAB Function3/2(Y)
  X2/1 -> MATLAB Function3/1(X)
  I/1 -> MATLAB Function/4(I)
  MATLAB Function/2(Hy_xp) -> MATLAB Function4/2(Hy_xp)
  MATLAB Function3/6(Hz_yn) -> MATLAB Function4/12(Hz_yn)
  MATLAB Function3/5(Hy_yn) -> MATLAB Function4/11(Hy_yn)
  MATLAB Function/5(Hy_xn) -> MATLAB Function4/5(Hy_xn)
  Y/1 -> MATLAB Function/2(Y)
  MATLAB Function3/2(Hy_yp) -> MATLAB Function4/8(Hy_yp)
  MATLAB Function/1(Hx_xp) -> MATLAB Function4/1(Hx_xp)
  MATLAB Function/4(Hx_xn) -> MATLAB Function4/4(Hx_xn)
  MATLAB Function3/3(Hz_yp) -> MATLAB Function4/9(Hz_yp)
  MATLAB Function3/4(Hx_yn) -> MATLAB Function4/10(Hx_yn)
  MATLAB Function3/1(Hx_yp) -> MATLAB Function4/7(Hx_yp)
  MATLAB Function4/2(Hy) -> Hy/1
  MATLAB Function/3(Hz_xp) -> MATLAB Function4/3(Hz_xp)
  Z/1 -> MATLAB Function/3(Z)
  MATLAB Function/6(Hz_xn) -> MATLAB Function4/6(Hz_xn)
  I1/1 -> MATLAB Function3/4(I)
  MATLAB Function4/1(Hx) -> Hx/1
  X/1 -> MATLAB Function/1(X)
  MATLAB Function4/3(Hz) -> Hz/1

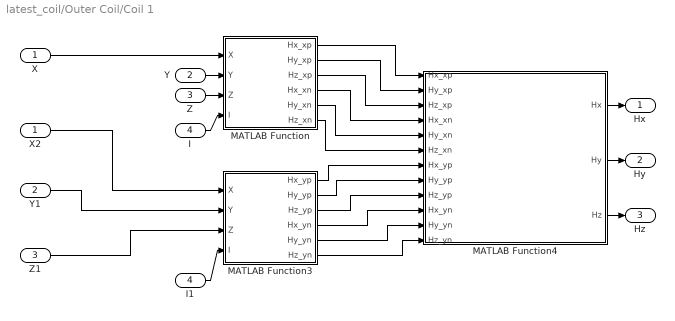
== system latest_coil/Outer Coil/Coil 1 ==
  X : Inport
  Y : Inport  Port=2
  Z : Inport  Port=3
  I : Inport  Port=4
  I1 : InportShadow  Port=4
  MATLAB Function : MATLAB Function  TreatAsAtomicUnit=on
  MATLAB Function3 : MATLAB Function  TreatAsAtomicUnit=on
  MATLAB Function4 : MATLAB Function  TreatAsAtomicUnit=on
  X2 : InportShadow
  Y1 : InportShadow  Port=2
  Z1 : InportShadow  Port=3
  Hx : Outport
  Hy : Outport  Port=2
  Hz : Outport  Port=3
  wires:
  Z1/1 -> MATLAB Function3/3(Z)
  Y1/1 -> MATLAB Function3/2(Y)
  X2/1 -> MATLAB Function3/1(X)
  I/1 -> MATLAB Function/4(I)
  MATLAB Function/2(Hy_xp) -> MATLAB Function4/2(Hy_xp)
  MATLAB Function3/6(Hz_yn) -> MATLAB Function4/12(Hz_yn)
  MATLAB Function3/5(Hy_yn) -> MATLAB Function4/11(Hy_yn)
  MATLAB Function/5(Hy_xn) -> MATLAB Function4/5(Hy_xn)
  Y/1 -> MATLAB Function/2(Y)
  MATLAB Function3/2(Hy_yp) -> MATLAB Function4/8(Hy_yp)
  MATLAB Function/1(Hx_xp) -> MATLAB Function4/1(Hx_xp)
  MATLAB Function/4(Hx_xn) -> MATLAB Function4/4(Hx_xn)
  MATLAB Function3/3(Hz_yp) -> MATLAB Function4/9(Hz_yp)
  MATLAB Function3/4(Hx_yn) -> MATLAB Function4/10(Hx_yn)
  MATLAB Function3/1(Hx_yp) -> MATLAB Function4/7(Hx_yp)
  MATLAB Function4/2(Hy) -> Hy/1
  MATLAB Function/3(Hz_xp) -> MATLAB Function4/3(Hz_xp)
  Z/1 -> MATLAB Function/3(Z)
  MATLAB Function/6(Hz_xn) -> MATLAB Function4/6(Hz_xn)
  I1/1 -> MATLAB Function3/4(I)
  MATLAB Function4/1(Hx) -> Hx/1
  X/1 -> MATLAB Function/1(X)
  MATLAB Function4/3(Hz) -> Hz/1

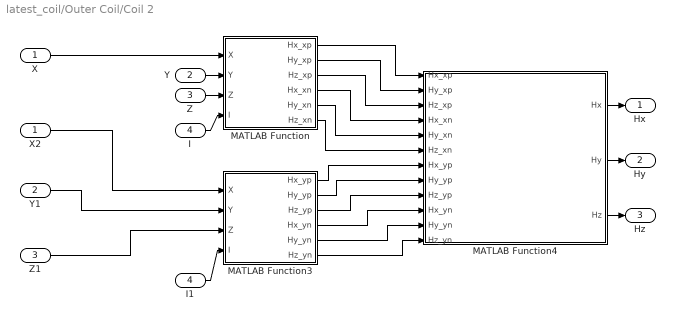
== system latest_coil/Outer Coil/Coil 2 ==
  X : Inport
  Y : Inport  Port=2
  Z : Inport  Port=3
  I : Inport  Port=4
  I1 : InportShadow  Port=4
  MATLAB Function : MATLAB Function  TreatAsAtomicUnit=on
  MATLAB Function3 : MATLAB Function  TreatAsAtomicUnit=on
  MATLAB Function4 : MATLAB Function  TreatAsAtomicUnit=on
  X2 : InportShadow
  Y1 : InportShadow  Port=2
  Z1 : InportShadow  Port=3
  Hx : Outport
  Hy : Outport  Port=2
  Hz : Outport  Port=3
  wires:
  MATLAB Function4/3(Hz) -> Hz/1
  X/1 -> MATLAB Function/1(X)
  MATLAB Function4/1(Hx) -> Hx/1
  I1/1 -> MATLAB Function3/4(I)
  MATLAB Function/6(Hz_xn) -> MATLAB Function4/6(Hz_xn)
  Z/1 -> MATLAB Function/3(Z)
  MATLAB Function/3(Hz_xp) -> MATLAB Function4/3(Hz_xp)
  MATLAB Function4/2(Hy) -> Hy/1
  MATLAB Function3/1(Hx_yp) -> MATLAB Function4/7(Hx_yp)
  MATLAB Function3/4(Hx_yn) -> MATLAB Function4/10(Hx_yn)
  MATLAB Function3/3(Hz_yp) -> MATLAB Function4/9(Hz_yp)
  MATLAB Function/4(Hx_xn) -> MATLAB Function4/4(Hx_xn)
  MATLAB Function/1(Hx_xp) -> MATLAB Function4/1(Hx_xp)
  MATLAB Function3/2(Hy_yp) -> MATLAB Function4/8(Hy_yp)
  Y/1 -> MATLAB Function/2(Y)
  MATLAB Function/5(Hy_xn) -> MATLAB Function4/5(Hy_xn)
  MATLAB Function3/5(Hy_yn) -> MATLAB Function4/11(Hy_yn)
  MATLAB Function3/6(Hz_yn) -> MATLAB Function4/12(Hz_yn)
  MATLAB Function/2(Hy_xp) -> MATLAB Function4/2(Hy_xp)
  I/1 -> MATLAB Function/4(I)
  X2/1 -> MATLAB Function3/1(X)
  Y1/1 -> MATLAB Function3/2(Y)
  Z1/1 -> MATLAB Function3/3(Z)

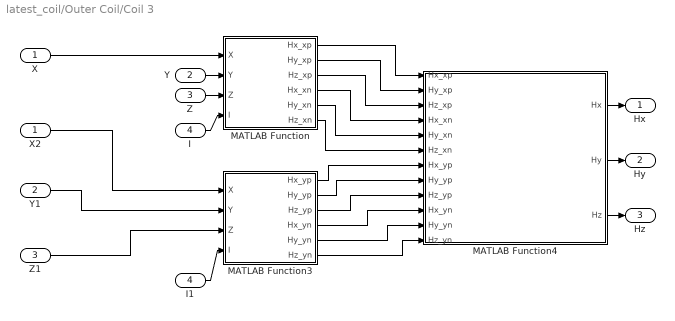
== system latest_coil/Outer Coil/Coil 3 ==
  X : Inport
  Y : Inport  Port=2
  Z : Inport  Port=3
  I : Inport  Port=4
  I1 : InportShadow  Port=4
  MATLAB Function : MATLAB Function  TreatAsAtomicUnit=on
  MATLAB Function3 : MATLAB Function  TreatAsAtomicUnit=on
  MATLAB Function4 : MATLAB Function  TreatAsAtomicUnit=on
  X2 : InportShadow
  Y1 : InportShadow  Port=2
  Z1 : InportShadow  Port=3
  Hx : Outport
  Hy : Outport  Port=2
  Hz : Outport  Port=3
  wires:
  MATLAB Function4/3(Hz) -> Hz/1
  X/1 -> MATLAB Function/1(X)
  MATLAB Function4/1(Hx) -> Hx/1
  I1/1 -> MATLAB Function3/4(I)
  MATLAB Function/6(Hz_xn) -> MATLAB Function4/6(Hz_xn)
  Z/1 -> MATLAB Function/3(Z)
  MATLAB Function/3(Hz_xp) -> MATLAB Function4/3(Hz_xp)
  MATLAB Function4/2(Hy) -> Hy/1
  MATLAB Function3/1(Hx_yp) -> MATLAB Function4/7(Hx_yp)
  MATLAB Function3/4(Hx_yn) -> MATLAB Function4/10(Hx_yn)
  MATLAB Function3/3(Hz_yp) -> MATLAB Function4/9(Hz_yp)
  MATLAB Function/4(Hx_xn) -> MATLAB Function4/4(Hx_xn)
  MATLAB Function/1(Hx_xp) -> MATLAB Function4/1(Hx_xp)
  MATLAB Function3/2(Hy_yp) -> MATLAB Function4/8(Hy_yp)
  Y/1 -> MATLAB Function/2(Y)
  MATLAB Function/5(Hy_xn) -> MATLAB Function4/5(Hy_xn)
  MATLAB Function3/5(Hy_yn) -> MATLAB Function4/11(Hy_yn)
  MATLAB Function3/6(Hz_yn) -> MATLAB Function4/12(Hz_yn)
  MATLAB Function/2(Hy_xp) -> MATLAB Function4/2(Hy_xp)
  I/1 -> MATLAB Function/4(I)
  X2/1 -> MATLAB Function3/1(X)
  Y1/1 -> MATLAB Function3/2(Y)
  Z1/1 -> MATLAB Function3/3(Z)

== system latest_coil/Outer Coil/Coil 4 ==
  X : Inport
  Y : Inport  Port=2
  Z : Inport  Port=3
  I : Inport  Port=4
  I1 : InportShadow  Port=4
  MATLAB Function : MATLAB Function  TreatAsAtomicUnit=on
  MATLAB Function3 : MATLAB Function  TreatAsAtomicUnit=on
  MATLAB Function4 : MATLAB Function  TreatAsAtomicUnit=on
  X2 : InportShadow
  Y1 : InportShadow  Port=2
  Z1 : InportShadow  Port=3
  Hx : Outport
  Hy : Outport  Port=2
  Hz : Outport  Port=3
  wires:
  Z1/1 -> MATLAB Function3/3(Z)
  Y1/1 -> MATLAB Function3/2(Y)
  X2/1 -> MATLAB Function3/1(X)
  I/1 -> MATLAB Function/4(I)
  MATLAB Function/2(Hy_xp) -> MATLAB Function4/2(Hy_xp)
  MATLAB Function3/6(Hz_yn) -> MATLAB Function4/12(Hz_yn)
  MATLAB Function3/5(Hy_yn) -> MATLAB Function4/11(Hy_yn)
  MATLAB Function/5(Hy_xn) -> MATLAB Function4/5(Hy_xn)
  Y/1 -> MATLAB Function/2(Y)
  MATLAB Function3/2(Hy_yp) -> MATLAB Function4/8(Hy_yp)
  MATLAB Function/1(Hx_xp) -> MATLAB Function4/1(Hx_xp)
  MATLAB Function/4(Hx_xn) -> MATLAB Function4/4(Hx_xn)
  MATLAB Function3/3(Hz_yp) -> MATLAB Function4/9(Hz_yp)
  MATLAB Function3/4(Hx_yn) -> MATLAB Function4/10(Hx_yn)
  MATLAB Function3/1(Hx_yp) -> MATLAB Function4/7(Hx_yp)
  MATLAB Function4/2(Hy) -> Hy/1
  MATLAB Function/3(Hz_xp) -> MATLAB Function4/3(Hz_xp)
  Z/1 -> MATLAB Function/3(Z)
  MATLAB Function/6(Hz_xn) -> MATLAB Function4/6(Hz_xn)
  I1/1 -> MATLAB Function3/4(I)
  MATLAB Function4/1(Hx) -> Hx/1
  X/1 -> MATLAB Function/1(X)
  MATLAB Function4/3(Hz) -> Hz/1

== system latest_coil/Outer Coil/Coil 5 ==
  X : Inport
  Y : Inport  Port=2
  Z : Inport  Port=3
  I : Inport  Port=4
  I1 : InportShadow  Port=4
  MATLAB Function : MATLAB Function  TreatAsAtomicUnit=on
  MATLAB Function3 : MATLAB Function  TreatAsAtomicUnit=on
  MATLAB Function4 : MATLAB Function  TreatAsAtomicUnit=on
  X2 : InportShadow
  Y1 : InportShadow  Port=2
  Z1 : InportShadow  Port=3
  Hx : Outport
  Hy : Outport  Port=2
  Hz : Outport  Port=3
  wires:
  MATLAB Function4/3(Hz) -> Hz/1
  X/1 -> MATLAB Function/1(X)
  MATLAB Function4/1(Hx) -> Hx/1
  I1/1 -> MATLAB Function3/4(I)
  MATLAB Function/6(Hz_xn) -> MATLAB Function4/6(Hz_xn)
  Z/1 -> MATLAB Function/3(Z)
  MATLAB Function/3(Hz_xp) -> MATLAB Function4/3(Hz_xp)
  MATLAB Function4/2(Hy) -> Hy/1
  MATLAB Function3/1(Hx_yp) -> MATLAB Function4/7(Hx_yp)
  MATLAB Function3/4(Hx_yn) -> MATLAB Function4/10(Hx_yn)
  MATLAB Function3/3(Hz_yp) -> MATLAB Function4/9(Hz_yp)
  MATLAB Function/4(Hx_xn) -> MATLAB Function4/4(Hx_xn)
  MATLAB Function/1(Hx_xp) -> MATLAB Function4/1(Hx_xp)
  MATLAB Function3/2(Hy_yp) -> MATLAB Function4/8(Hy_yp)
  Y/1 -> MATLAB Function/2(Y)
  MATLAB Function/5(Hy_xn) -> MATLAB Function4/5(Hy_xn)
  MATLAB Function3/5(Hy_yn) -> MATLAB Function4/11(Hy_yn)
  MATLAB Function3/6(Hz_yn) -> MATLAB Function4/12(Hz_yn)
  MATLAB Function/2(Hy_xp) -> MATLAB Function4/2(Hy_xp)
  I/1 -> MATLAB Function/4(I)
  X2/1 -> MATLAB Function3/1(X)
  Y1/1 -> MATLAB Function3/2(Y)
  Z1/1 -> MATLAB Function3/3(Z)

== matlab function latest_coil/Inner Coil/Coil 2/MATLAB Function3 ==
  data: X input; Hx_yp output; Y input; Z input; I input; Hy_yp output; Hz_yp output; Hx_yn output; Hy_yn output; Hz_yn output
function [Hx_yp, Hy_yp, Hz_yp, Hx_yn, Hy_yn, Hz_yn] = field_y(X, Y, Z, I)
n = 1;
gy = 520e-6;
% gx = 675e-6;
gz = 0;
m0 = 4*pi*1e-7;
k = 0.4e-3;
yp1 = -0.6e-3 - (n-1)*k;
yp2 = 0.6e-3 + (n-1)*k;
a_xp = gy;
a_zp = gz;
k_yp = 1./(4*pi*((a_xp-X).^2+(a_zp-Z).^2));
kyp = (yp2-Y)./((yp2-Y).^2+(a_xp-X).^2+(a_zp-Z).^2).^0.5;
k_2yp = (yp1-Y)./((yp1-Y).^2+(a_xp-X).^2+(a_zp-Z).^2).^0.5;

Hx_yp = -((a_zp-Z).*k_yp.*(kyp - k_2yp))*I*m0;
Hy_yp = zeros(size(X,1),size(Y,1),size(Z,1));
Hz_yp = (-(a_xp-X).*k_yp.*(kyp - k_2yp))*I*m0;

a_xn = -gy;
yn1 = -0.8e-3 - (n-1)*k;
yn2 = 0.8e-3 + (n-1)*k;
k_yn = 1./(4*pi*((a_xn-X).^2+(a_zp-Z).^2));
kyn = (yn2-Y)./((yn2-Y).^2+(a_xn-X).^2+(a_zp-Z).^2).^0.5;
k_2yn = (yn1-Y)./((yn1-Y).^2+(a_xn-X).^2+(a_zp-Z).^2).^0.5;

Hx_yn = ((a_zp-Z).*k_yn.*(kyn - k_2yn))*I*m0;
Hy_yn = zeros(size(X,1),size(Y,1),size(Z,1));
Hz_yn = ((a_xn-X).*k_yn.*(kyn - k_2yn))*I*m0;

end

== matlab function latest_coil/Inner Coil/Coil 2/MATLAB Function4 ==
  data: Hx_xp input; Hy_xp input; Hz_xp input; Hx output; Hx_xn input; Hy_xn input; Hy output; Hz output; Hz_xn input; Hx_yp input; Hy_yp input; Hz_yp input; Hx_yn input; Hy_yn input; Hz_yn input
function [Hx, Hy, Hz] = field_sum(Hx_xp, Hy_xp, Hz_xp, Hx_xn, Hy_xn, Hz_xn, Hx_yp, Hy_yp, Hz_yp, Hx_yn, Hy_yn, Hz_yn)
Hx = Hx_xp + Hx_xn + Hx_yp + Hx_yn;
Hy = Hy_xp + Hy_xn + Hy_yp + Hy_yn;
Hz = Hz_xp + Hz_xn + Hz_yp + Hz_yn;
end

== matlab function latest_coil/MATLAB Function1 ==
  data: Ff_y output; Fext_y input; vy input
function Ff_y = friction(Fext_y,vy)
Coeff_of_Fric = 0.432;
g = 9.8;
mass_of_bot = 9.17345e-05;

% if  Fext_y < 0 && vy >= 0 %When force is in negative direction and velocity is in positive direction (impossible case) (Removing this case implies object doesn't move)
%     Ff_y = 0;
% elseif  Fext_y > 0 && vy <= 0 %When force is in positivedirection and velocity is in positive direction (impossible case)
%     Ff_y = 0;
% elseif  vy < 0 %When velocity is in negative direction friction is positive (Object is moving)
%     Ff_y = Coeff_of_Fric*mass_of_bot*g;
% elseif  vy > 0 %When velocity is in positive direction friction is negative (Object is moving)
%     Ff_y = -Coeff_of_Fric*mass_of_bot*g;
% elseif (abs(Fext_y) >= Coeff_of_Fric*mass_of_bot*g  &&  vy < 0 ) || (abs(Fext_y) >= Coeff_of_Fric*mass_of_bot*g && vy > 0) %When applied force greater than couloumb friction and 
%                                                                                                                        % moves is positive or negative direction, then Couloumb friction opposes that motion
%     Ff_y = -Coeff_of_Fric*mass_of_bot*g*sign(Fext_y);
% 
% elseif (abs(Fext_y) < Coeff_of_Fric*mass_of_bot*g && Fext_y~= 0) %When applied force less than Coloumb Friction but not equal to zero, Friction force is applied force
%     Ff_y = -Fext_y;
% else %When applied force is zero or when object not moving
%     Ff_y = -Fext_y;
% end

if abs(vy)<0.01
    if abs(Fext_y)>Coeff_of_Fric*mass_of_bot*g
        Ff_y=-Coeff_of_Fric*mass_of_bot*g*sign(Fext_y);
    else
        Ff_y=-Fext_y-vy;
    end
else
    Ff_y=-Coeff_of_Fric*mass_of_bot*g*sign(vy);
end

== matlab function latest_coil/Inner Coil/Coil 3/MATLAB Function ==
  data: X input; Hx_xp output; Y input; Z input; I input; Hy_xp output; Hz_xp output; Hx_xn output; Hy_xn output; Hz_xn output
function [Hx_xp, Hy_xp, Hz_xp, Hx_xn, Hy_xn, Hz_xn] = field_x(X, Y, Z, I)
n = 1;
gx = 675e-6;
gz = 0;
m0 = 4*pi*1e-7;
k = 0.4e-3;
xp_1 = -0.8e-3 - (n-1)*k;
xp_2 = 0.8e-3 + (n-1)*k;
a_yp = gx; 
a_zp = gz;
k_p = 1./(4*pi*((a_yp-Y).^2+(a_zp-Z).^2));
kxp = (xp_2-X)./((xp_2-X).^2+(a_yp-Y).^2+(a_zp-Z).^2).^0.5;
k_2xp = (xp_1-X)./((xp_1-X).^2+(a_yp-Y).^2+(a_zp-Z).^2).^0.5;

Hx_xp = zeros(size(X,1),size(Y,1),size(Z,1));
Hy_xp = (-(a_zp-Z).*k_p.*(kxp - k_2xp))*I*m0;
Hz_xp = (-(a_yp-Y).*k_p.*(kxp - k_2xp))*I*m0;

a_yn = -gx;
xn_1 = -1e-3 - (n-1)*k;
xn_2 = 1e-3 + (n-1)*k;
k_n = 1./(4*pi*((a_yn-Y).^2+(a_zp-Z).^2));
kxn = (xn_2-X)./((xn_2-X).^2+(a_yn-Y).^2+(a_zp-Z).^2).^0.5;
k_2xn = (xn_1-X)./((xn_1-X).^2+(a_yn-Y).^2+(a_zp-Z).^2).^0.5;

Hx_xn = zeros(size(X,1),size(Y,1),size(Z,1));
Hy_xn = ((a_zp-Z).*k_n.*(kxn - k_2xn))*I*m0;
Hz_xn = ((a_yn-Y).*k_n.*(kxn - k_2xn))*I*m0;

end

== matlab function latest_coil/Inner Coil/Coil 3/MATLAB Function3 ==
  data: X input; Hx_yp output; Y input; Z input; I input; Hy_yp output; Hz_yp output; Hx_yn output; Hy_yn output; Hz_yn output
function [Hx_yp, Hy_yp, Hz_yp, Hx_yn, Hy_yn, Hz_yn] = field_y(X, Y, Z, I)
n = 1;
gy = 520e-6;
% gx = 675e-6;
gz = 0;
m0 = 4*pi*1e-7;
k = 0.4e-3;
yp1 = -0.6e-3 - (n-1)*k;
yp2 = 0.6e-3 - (n-1)*k;
a_xp = gy;
a_zp = gz;
k_yp = 1./(4*pi*((a_xp-X).^2+(a_zp-Z).^2));
kyp = (yp2-Y)./((yp2-Y).^2+(a_xp-X).^2+(a_zp-Z).^2).^0.5;
k_2yp = (yp1-Y)./((yp1-Y).^2+(a_xp-X).^2+(a_zp-Z).^2).^0.5;

Hx_yp = -((a_zp-Z).*k_yp.*(kyp - k_2yp))*I*m0;
Hy_yp = zeros(size(X,1),size(Y,1),size(Z,1));
Hz_yp = (-(a_xp-X).*k_yp.*(kyp - k_2yp))*I*m0;

a_xn = -gy;
yn1 = -0.8e-3 - (n-1)*k;
yn2 = 0.8e-3 - (n-1)*k;
k_yn = 1./(4*pi*((a_xn-X).^2+(a_zp-Z).^2));
kyn = (yn2-Y)./((yn2-Y).^2+(a_xn-X).^2+(a_zp-Z).^2).^0.5;
k_2yn = (yn1-Y)./((yn1-Y).^2+(a_xn-X).^2+(a_zp-Z).^2).^0.5;

Hx_yn = ((a_zp-Z).*k_yn.*(kyn - k_2yn))*I*m0;
Hy_yn = zeros(size(X,1),size(Y,1),size(Z,1));
Hz_yn = ((a_xn-X).*k_yn.*(kyn - k_2yn))*I*m0;

end

== matlab function latest_coil/Inner Coil/Coil 3/MATLAB Function4 ==
  data: Hx_xp input; Hy_xp input; Hz_xp input; Hx output; Hx_xn input; Hy_xn input; Hy output; Hz output; Hz_xn input; Hx_yp input; Hy_yp input; Hz_yp input; Hx_yn input; Hy_yn input; Hz_yn input
function [Hx, Hy, Hz] = field_sum(Hx_xp, Hy_xp, Hz_xp, Hx_xn, Hy_xn, Hz_xn, Hx_yp, Hy_yp, Hz_yp, Hx_yn, Hy_yn, Hz_yn)
Hx = Hx_xp + Hx_xn + Hx_yp + Hx_yn;
Hy = Hy_xp + Hy_xn + Hy_yp + Hy_yn;
Hz = Hz_xp + Hz_xn + Hz_yp + Hz_yn;
end

== matlab function latest_coil/Inner Coil/Coil 4/MATLAB Function ==
  data: X input; Hx_xp output; Y input; Z input; I input; Hy_xp output; Hz_xp output; Hx_xn output; Hy_xn output; Hz_xn output
function [Hx_xp, Hy_xp, Hz_xp, Hx_xn, Hy_xn, Hz_xn] = field_x(X, Y, Z, I)
n = 1;
gx = 675e-6;
gz = 0;
m0 = 4*pi*1e-7;
k = 0.4e-3;
xp_1 = -0.8e-3 - (n-1)*k;
xp_2 = 0.8e-3 + (n-1)*k;
a_yp = gx; 
a_zp = gz;
k_p = 1./(4*pi*((a_yp-Y).^2+(a_zp-Z).^2));
kxp = (xp_2-X)./((xp_2-X).^2+(a_yp-Y).^2+(a_zp-Z).^2).^0.5;
k_2xp = (xp_1-X)./((xp_1-X).^2+(a_yp-Y).^2+(a_zp-Z).^2).^0.5;

Hx_xp = zeros(size(X,1),size(Y,1),size(Z,1));
Hy_xp = (-(a_zp-Z).*k_p.*(kxp - k_2xp))*I*m0;
Hz_xp = (-(a_yp-Y).*k_p.*(kxp - k_2xp))*I*m0;

a_yn = -gx;
xn_1 = -1e-3 - (n-1)*k;
xn_2 = 1e-3 + (n-1)*k;
k_n = 1./(4*pi*((a_yn-Y).^2+(a_zp-Z).^2));
kxn = (xn_2-X)./((xn_2-X).^2+(a_yn-Y).^2+(a_zp-Z).^2).^0.5;
k_2xn = (xn_1-X)./((xn_1-X).^2+(a_yn-Y).^2+(a_zp-Z).^2).^0.5;

Hx_xn = zeros(size(X,1),size(Y,1),size(Z,1));
Hy_xn = ((a_zp-Z).*k_n.*(kxn - k_2xn))*I*m0;
Hz_xn = ((a_yn-Y).*k_n.*(kxn - k_2xn))*I*m0;

end

== matlab function latest_coil/Inner Coil/Coil 4/MATLAB Function3 ==
  data: X input; Hx_yp output; Y input; Z input; I input; Hy_yp output; Hz_yp output; Hx_yn output; Hy_yn output; Hz_yn output
function [Hx_yp, Hy_yp, Hz_yp, Hx_yn, Hy_yn, Hz_yn] = field_y(X, Y, Z, I)
n = 1;
gy = 520e-6;
% gx = 675e-6;
gz = 0;
m0 = 4*pi*1e-7;
k = 0.4e-3;
yp1 = -0.6e-3 - (n-1)*k;
yp2 = 0.6e-3 - (n-1)*k;
a_xp = gy;
a_zp = gz;
k_yp = 1./(4*pi*((a_xp-X).^2+(a_zp-Z).^2));
kyp = (yp2-Y)./((yp2-Y).^2+(a_xp-X).^2+(a_zp-Z).^2).^0.5;
k_2yp = (yp1-Y)./((yp1-Y).^2+(a_xp-X).^2+(a_zp-Z).^2).^0.5;

Hx_yp = -((a_zp-Z).*k_yp.*(kyp - k_2yp))*I*m0;
Hy_yp = zeros(size(X,1),size(Y,1),size(Z,1));
Hz_yp = (-(a_xp-X).*k_yp.*(kyp - k_2yp))*I*m0;

a_xn = -gy;
yn1 = -0.8e-3 - (n-1)*k;
yn2 = 0.8e-3 - (n-1)*k;
k_yn = 1./(4*pi*((a_xn-X).^2+(a_zp-Z).^2));
kyn = (yn2-Y)./((yn2-Y).^2+(a_xn-X).^2+(a_zp-Z).^2).^0.5;
k_2yn = (yn1-Y)./((yn1-Y).^2+(a_xn-X).^2+(a_zp-Z).^2).^0.5;

Hx_yn = ((a_zp-Z).*k_yn.*(kyn - k_2yn))*I*m0;
Hy_yn = zeros(size(X,1),size(Y,1),size(Z,1));
Hz_yn = ((a_xn-X).*k_yn.*(kyn - k_2yn))*I*m0;

end

== matlab function latest_coil/Inner Coil/Coil 4/MATLAB Function4 ==
  data: Hx_xp input; Hy_xp input; Hz_xp input; Hx output; Hx_xn input; Hy_xn input; Hy output; Hz output; Hz_xn input; Hx_yp input; Hy_yp input; Hz_yp input; Hx_yn input; Hy_yn input; Hz_yn input
function [Hx, Hy, Hz] = field_sum(Hx_xp, Hy_xp, Hz_xp, Hx_xn, Hy_xn, Hz_xn, Hx_yp, Hy_yp, Hz_yp, Hx_yn, Hy_yn, Hz_yn)
Hx = Hx_xp + Hx_xn + Hx_yp + Hx_yn;
Hy = Hy_xp + Hy_xn + Hy_yp + Hy_yn;
Hz = Hz_xp + Hz_xn + Hz_yp + Hz_yn;
end

== matlab function latest_coil/Inner Coil/Coil 5/MATLAB Function ==
  data: X input; Hx_xp output; Y input; Z input; I input; Hy_xp output; Hz_xp output; Hx_xn output; Hy_xn output; Hz_xn output
function [Hx_xp, Hy_xp, Hz_xp, Hx_xn, Hy_xn, Hz_xn] = field_x(X, Y, Z, I)
n = 1;
gx = 675e-6;
gz = 0;
m0 = 4*pi*1e-7;
k = 0.4e-3;
xp_1 = -0.8e-3 - (n-1)*k;
xp_2 = 0.8e-3 + (n-1)*k;
a_yp = gx; 
a_zp = gz;
k_p = 1./(4*pi*((a_yp-Y).^2+(a_zp-Z).^2));
kxp = (xp_2-X)./((xp_2-X).^2+(a_yp-Y).^2+(a_zp-Z).^2).^0.5;
k_2xp = (xp_1-X)./((xp_1-X).^2+(a_yp-Y).^2+(a_zp-Z).^2).^0.5;

Hx_xp = zeros(size(X,1),size(Y,1),size(Z,1));
Hy_xp = (-(a_zp-Z).*k_p.*(kxp - k_2xp))*I*m0;
Hz_xp = (-(a_yp-Y).*k_p.*(kxp - k_2xp))*I*m0;

a_yn = -gx;
xn_1 = -1e-3 - (n-1)*k;
xn_2 = 1e-3 + (n-1)*k;
k_n = 1./(4*pi*((a_yn-Y).^2+(a_zp-Z).^2));
kxn = (xn_2-X)./((xn_2-X).^2+(a_yn-Y).^2+(a_zp-Z).^2).^0.5;
k_2xn = (xn_1-X)./((xn_1-X).^2+(a_yn-Y).^2+(a_zp-Z).^2).^0.5;

Hx_xn = zeros(size(X,1),size(Y,1),size(Z,1));
Hy_xn = ((a_zp-Z).*k_n.*(kxn - k_2xn))*I*m0;
Hz_xn = ((a_yn-Y).*k_n.*(kxn - k_2xn))*I*m0;

end

== matlab function latest_coil/Inner Coil/Coil 5/MATLAB Function3 ==
  data: X input; Hx_yp output; Y input; Z input; I input; Hy_yp output; Hz_yp output; Hx_yn output; Hy_yn output; Hz_yn output
function [Hx_yp, Hy_yp, Hz_yp, Hx_yn, Hy_yn, Hz_yn] = field_y(X, Y, Z, I)
n = 1;
gy = 520e-6;
% gx = 675e-6;
gz = 0;
m0 = 4*pi*1e-7;
k = 0.4e-3;
yp1 = -0.6e-3 - (n-1)*k;
yp2 = 0.6e-3 - (n-1)*k;
a_xp = gy;
a_zp = gz;
k_yp = 1./(4*pi*((a_xp-X).^2+(a_zp-Z).^2));
kyp = (yp2-Y)./((yp2-Y).^2+(a_xp-X).^2+(a_zp-Z).^2).^0.5;
k_2yp = (yp1-Y)./((yp1-Y).^2+(a_xp-X).^2+(a_zp-Z).^2).^0.5;

Hx_yp = -((a_zp-Z).*k_yp.*(kyp - k_2yp))*I*m0;
Hy_yp = zeros(size(X,1),size(Y,1),size(Z,1));
Hz_yp = (-(a_xp-X).*k_yp.*(kyp - k_2yp))*I*m0;

a_xn = -gy;
yn1 = -0.8e-3 - (n-1)*k;
yn2 = 0.8e-3 - (n-1)*k;
k_yn = 1./(4*pi*((a_xn-X).^2+(a_zp-Z).^2));
kyn = (yn2-Y)./((yn2-Y).^2+(a_xn-X).^2+(a_zp-Z).^2).^0.5;
k_2yn = (yn1-Y)./((yn1-Y).^2+(a_xn-X).^2+(a_zp-Z).^2).^0.5;

Hx_yn = ((a_zp-Z).*k_yn.*(kyn - k_2yn))*I*m0;
Hy_yn = zeros(size(X,1),size(Y,1),size(Z,1));
Hz_yn = ((a_xn-X).*k_yn.*(kyn - k_2yn))*I*m0;

end

== matlab function latest_coil/Inner Coil/Coil 5/MATLAB Function4 ==
  data: Hx_xp input; Hy_xp input; Hz_xp input; Hx output; Hx_xn input; Hy_xn input; Hy output; Hz output; Hz_xn input; Hx_yp input; Hy_yp input; Hz_yp input; Hx_yn input; Hy_yn input; Hz_yn input
function [Hx, Hy, Hz] = field_sum(Hx_xp, Hy_xp, Hz_xp, Hx_xn, Hy_xn, Hz_xn, Hx_yp, Hy_yp, Hz_yp, Hx_yn, Hy_yn, Hz_yn)
Hx = Hx_xp + Hx_xn + Hx_yp + Hx_yn;
Hy = Hy_xp + Hy_xn + Hy_yp + Hy_yn;
Hz = Hz_xp + Hz_xn + Hz_yp + Hz_yn;
end

== matlab function latest_coil/Inner Coil/Coil 1/MATLAB Function3 ==
  data: X input; Hx_yp output; Y input; Z input; I input; Hy_yp output; Hz_yp output; Hx_yn output; Hy_yn output; Hz_yn output; dBx_dx output; dBx_dz output
function [Hx_yp, Hy_yp, Hz_yp, Hx_yn, Hy_yn, Hz_yn, dBx_dx, dBx_dz] = field_y(X, Y, Z, I)

== matlab function latest_coil/Outer Coil/Coil 1/MATLAB Function ==
  data: X input; Hx_xp output; Y input; Z input; I input; Hy_xp output; Hz_xp output; Hx_xn output; Hy_xn output; Hz_xn output
function [Hx_xp, Hy_xp, Hz_xp, Hx_xn, Hy_xn, Hz_xn] = field_x(X, Y, Z, I)
n = 1;
gx = 675e-6;
gz = 0;
m0 = 4*pi*1e-7;
k = 0.4e-3;
xp_1 = -0.8e-3 - (n-1)*k;
xp_2 = 0.8e-3 + (n-1)*k;
a_yp = gx; 
a_zp = gz;
k_p = 1./(4*pi*((a_yp-Y).^2+(a_zp-Z).^2));
kxp = (xp_2-X)./((xp_2-X).^2+(a_yp-Y).^2+(a_zp-Z).^2).^0.5;
k_2xp = (xp_1-X)./((xp_1-X).^2+(a_yp-Y).^2+(a_zp-Z).^2).^0.5;

Hx_xp = zeros(size(X,1),size(Y,1),size(Z,1));
Hy_xp = (-(a_zp-Z).*k_p.*(kxp - k_2xp))*I*m0;
Hz_xp = (-(a_yp-Y).*k_p.*(kxp - k_2xp))*I*m0;

a_yn = -gx;
xn_1 = -1e-3 - (n-1)*k;
xn_2 = 1e-3 + (n-1)*k;
k_n = 1./(4*pi*((a_yn-Y).^2+(a_zp-Z).^2));
kxn = (xn_2-X)./((xn_2-X).^2+(a_yn-Y).^2+(a_zp-Z).^2).^0.5;
k_2xn = (xn_1-X)./((xn_1-X).^2+(a_yn-Y).^2+(a_zp-Z).^2).^0.5;

Hx_xn = zeros(size(X,1),size(Y,1),size(Z,1));
Hy_xn = ((a_zp-Z).*k_n.*(kxn - k_2xn))*I*m0;
Hz_xn = ((a_yn-Y).*k_n.*(kxn - k_2xn))*I*m0;

end
